simulink model "Lab2_2_sim"  (R2016b)
settings: Solver=VariableStepAuto  StartTime=0.0  StopTime=0.1  RelTol=1e-3  EnableMultiTasking=on
settings Model: Creator=Yash Bansod  LastModifiedBy=Yash Bansod
settings DataIOCC: LimitDataPoints=on
settings OptimizationCC: LifeSpan=inf
settings DebuggingCC: AllowSymbolicDim=off  SFUnexpectedBacktrackingDiag=warning  SFNoUnconditionalDefaultTransitionDiag=warning  SFExecutionAtInitializationDiag=none
settings ModelReferenceCC: PropagateSignalLabelsOutOfModel=off
settings GRTTargetCC: TargetLangStandard=C89/C90 (ANSI)
settings ConfigComp: CovMetricSettings=dw  CovHtmlReporting=on  CovSaveCumulativeToWorkspaceVar=on  CovSaveSingleToWorkspaceVar=on  CovExternalEMLEnable=off

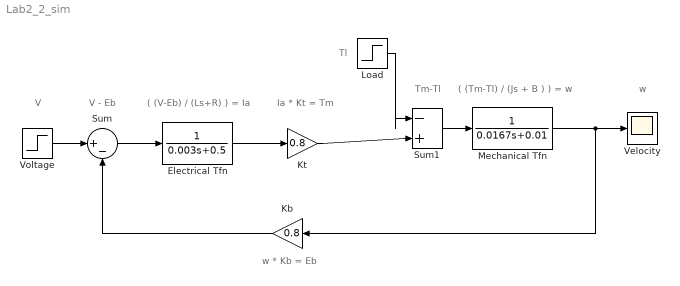
== system Lab2_2_sim ==
  note: Tm-Tl
  note: Tl
  note: V
  note: V - Eb
  note: ( (V-Eb) / (Ls+R) ) = Ia
  note: Ia * Kt = Tm
  note: ( (Tm-Tl) / (Js + B ) ) = w
  note: w
  note: w * Kb = Eb
  Electrical Tfn : TransferFcn  Denominator=[0.003 0.5]
  Kb : Gain  Gain=0.8
  Kt : Gain  Gain=0.8
  Load : Step  Time=0.015  After=100  SampleTime=0
  "Mechanical Tfn " : TransferFcn  Denominator=[0.0167 0.01]
  Sum : Sum  Inputs=|+-
  Sum1 : Sum  Inputs=|-+
  Velocity : Scope
  Voltage : Step  Time=0  After=220  SampleTime=0
  wires:
  Sum/1 -> Electrical Tfn/1
  Voltage/1 -> Sum/1
  Electrical Tfn/1 -> Kt/1
  "Mechanical Tfn "/1 -> Kb/1, Velocity/1
  Kb/1 -> Sum/2
  Sum1/1 -> "Mechanical Tfn "/1
  Kt/1 -> Sum1/2
  Load/1 -> Sum1/1
